simulink model "ex7"  (R2018a)
settings: Solver=VariableStepAuto  StartTime=0.0  StopTime=60  RelTol=1e-5
settings Model: Creator=HUAWEI  LastModifiedBy=HUAWEI

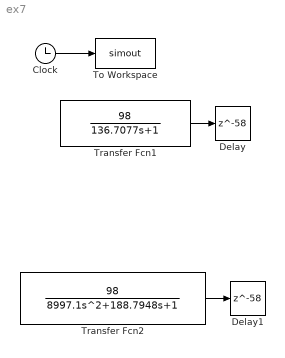
== system ex7 ==
  Clock : Clock
  Delay : Delay  DelayLength=58  InitialCondition=0
  Delay1 : Delay  DelayLength=58  InitialCondition=0
  To Workspace : ToWorkspace  VariableName=simout  SaveFormat=Timeseries  SampleTime=-1
  Transfer Fcn1 : TransferFcn  Numerator=[98]  Denominator=[136.7077 1]
  Transfer Fcn2 : TransferFcn  Numerator=[98]  Denominator=[8997.1 188.7948 1]
  wires:
  Clock/1 -> To Workspace/1
  Transfer Fcn1/1 -> Delay/1
  Transfer Fcn2/1 -> Delay1/1
